simulink model "Tema3_radial_dynamics"  (R2022b)
settings: Solver=ode4  StartTime=0.0  StopTime=4*pi  FixedStep=0.01  RelTol=1e-3
settings Model: Creator=scpmoxxa  LastModifiedBy=scpmoxxa

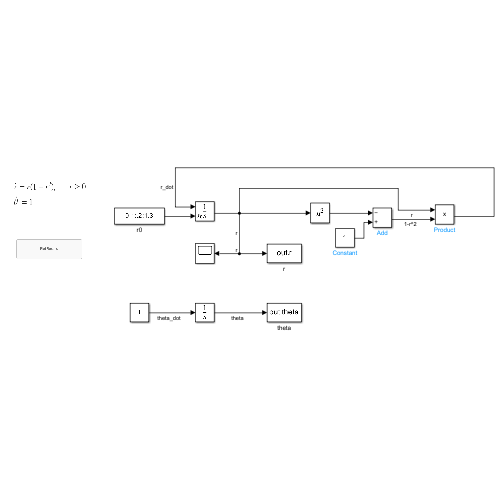
[thumbnail: Simulink's stored preview of the top-level diagram]
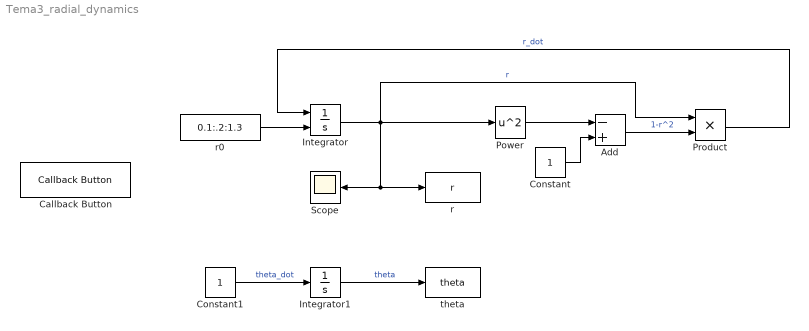
== system Tema3_radial_dynamics ==
  Add : Sum  Inputs=-+
  Callback Button : CallbackButton  ButtonText=Plot Results
      settings: ClickFcn=|
      | close all;
      | 
      | r = out.r;
      | theta = out.theta;
      | 
      | x = r .* cos(theta);
      | y = r .* sin(theta);
      | 
      | figure;
      | % Visualizar el espacio de fase
      | plot(x(:,1), y(:,1), 'LineWidth', 2);hold on
      | plot(x(:,2:end), y(:,2:end))
      | xlabel('x');
      | ylabel('y');
      | title('Limit Cycle');
      | axis square
  Constant : Constant
  Constant1 : Constant
  Integrator : Integrator  InitialConditionSource=external  InitialCondition=0.1
  Integrator1 : Integrator
  Power : Math  Operator=square
  Product : Product
  Scope : Scope
  r : ToWorkspace  VariableName=r  SampleTime=-1
  r0 : Constant  Value=0.1:.2:1.3
  theta : ToWorkspace  VariableName=theta  SampleTime=-1
  wires:
  Integrator/1 -> r/1, Scope/1, Power/1, Product/1  "r"
  Add/1 -> Product/2  "1-r^2"
  Product/1 -> Integrator/1  "r_dot"
  Constant1/1 -> Integrator1/1  "theta_dot"
  Integrator1/1 -> theta/1  "theta"
  Power/1 -> Add/1
  Constant/1 -> Add/2
  r0/1 -> Integrator/2
